simulink model "ME419_Ex1_4"  (R2023b)
settings: Solver=VariableStepAuto  StartTime=0.0  StopTime=10.0  RelTol=1e-3
settings Model: Creator=aliawolken  LastModifiedBy=aliawolken

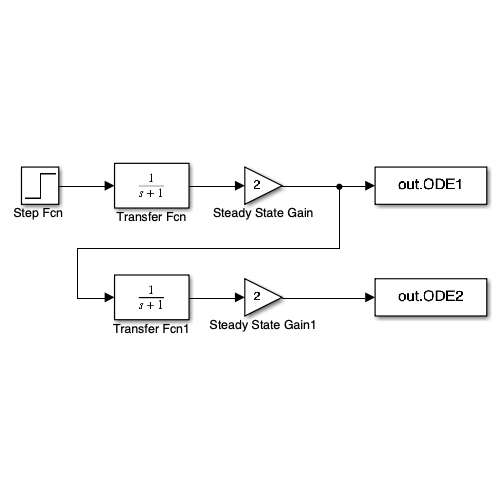
[thumbnail: Simulink's stored preview of the top-level diagram]
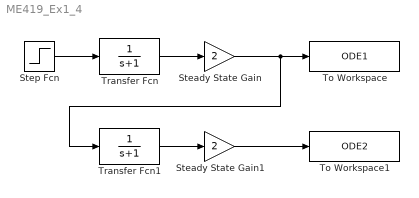
== system ME419_Ex1_4 ==
  Steady State Gain : Gain  Gain=2
  Steady State Gain1 : Gain  Gain=2
  "Step Fcn " : Step  SampleTime=0
  To Workspace : ToWorkspace  VariableName=ODE1  SaveFormat=Timeseries  SampleTime=-1
  To Workspace1 : ToWorkspace  VariableName=ODE2  SaveFormat=Timeseries  SampleTime=-1
  Transfer Fcn : TransferFcn  Denominator=[1 1]
  Transfer Fcn1 : TransferFcn  Denominator=[1 1]
  wires:
  "Step Fcn "/1 -> Transfer Fcn/1
  Transfer Fcn/1 -> Steady State Gain/1
  Transfer Fcn1/1 -> Steady State Gain1/1
  Steady State Gain1/1 -> To Workspace1/1
  Steady State Gain/1 -> To Workspace/1, Transfer Fcn1/1
